simulink model "MSE452_Lab3_PMSM_ForStudent_Finalv2"  (R2023a)
settings: Solver=ode45  StartTime=0.0  StopTime=0.3  MaxStep=1e-5  RelTol=1e-3  EnableMultiTasking=on
InitFcn:
  | Idc=0;
  | Vabc=0;
  | Iw=0;
values from neighbouring files (symbols this model uses):
  Flux = 0.7213*BaseFlux    [MSE452_Lab3_parameters.m]
  Ld = 0.7029*Lb    [MSE452_Lab3_parameters.m]
  Lq = 0.7029*Lb    [MSE452_Lab3_parameters.m]
  OMEGAb_r = OMEGAb/Ppairs    (= 41.885284054)    [MSE452_Lab3_parameters.m]
  Ppairs = 8    [MSE452_Lab3_parameters.m]
  RL = 1.2 * R    [MSE452_Lab3_parameters.m]
  Rs = 0.00517*Zb    [MSE452_Lab3_parameters.m]
undefined symbols (not defined in the file or in its folder): Ts
libraries: spspowerguiLib x1
settings Model: Creator=Administrator  LastModifiedBy=mitch
settings SolverCC: ZeroCrossControl=DisableAll  AlgebraicLoopSolver=TrustRegion
settings DataIOCC: LimitDataPoints=on  SaveFormat=Array  SignalLoggingSaveFormat=ModelDataLogs  ReturnWorkspaceOutputs=off
settings OptimizationCC: BlockReduction=off  DefaultParameterBehavior=Inlined  BufferReuse=off  ExpressionDepthLimit=2147483647  InitFltsAndDblsToZero=on  LifeSpan=inf
settings DebuggingCC: SaveWithParameterizedLinksMsg=none  UnderspecifiedInitializationDetection=Classic  MergeDetectMultiDrivingBlocksExec=none  SignalResolutionControl=TryResolveAllWithWarning  SolverPrmCheckMsg=warning  MultiTaskDSMMsg=warning  MultiTaskCondExecSysMsg=none  FcnCallInpInsideContextMsg=warning  UnconnectedInputMsg=warning  UnconnectedOutputMsg=warning  UnconnectedLineMsg=warning  StateNameClashWarn=warning  SFUnexpectedBacktrackingDiag=warning  SFNoUnconditionalDefaultTransitionDiag=warning  SFExecutionAtInitializationDiag=none  ArithmeticOperatorsInVariantConditions=warning
settings HardwareCC: ProdBitPerPointer=32  ProdBitPerSizeT=32  ProdBitPerPtrDiffT=32  ProdLargestAtomicFloat=None  ProdIntDivRoundTo=Undefined  ProdEndianess=Unspecified  ProdWordSize=32  ProdHWDeviceType=32-bit Generic
settings ModelReferenceCC: PropagateSignalLabelsOutOfModel=off
settings SFSimCC: SimUseLocalCustomCode=off  CustomCodeUndefinedFunction=UseInterfaceOnly
settings RTWCC: RTWUseLocalCustomCode=off
settings CodeAppCC: StateflowObjectComments=on
settings GRTTargetCC: TargetFcnLib=ansi_tfl_tmw.mat  TargetLangStandard=C89/C90 (ANSI)  CombineOutputUpdateFcns=off  GRTInterface=on
settings ConfigComp: CovMetricSettings=dw  CovSaveCumulativeToWorkspaceVar=on  CovSaveSingleToWorkspaceVar=on  CovExternalEMLEnable=off

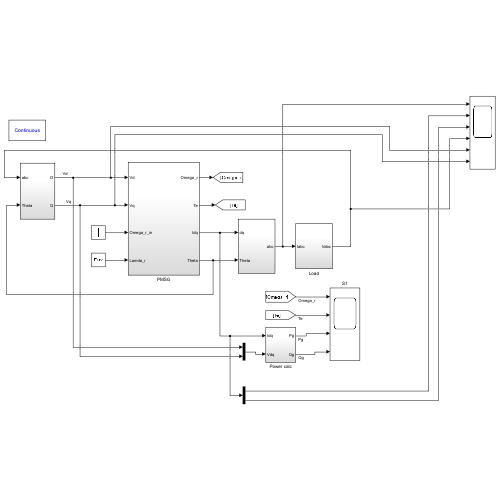
[thumbnail: Simulink's stored preview of the top-level diagram]
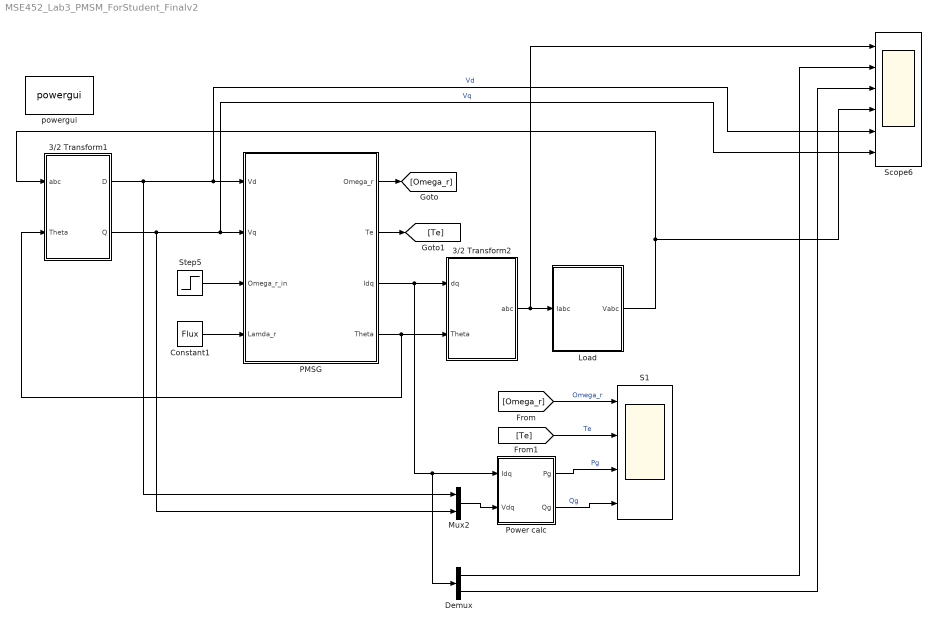
== system MSE452_Lab3_PMSM_ForStudent_Finalv2 ==
  3/2 Transform1 : Subsystem
  3/2 Transform2 : Subsystem
  Constant1 : Constant  Value=Flux
  Demux : Demux  Outputs=2
  Load : Subsystem
  Mux2 : Mux  Inputs=2
  PMSG : Subsystem
  Power calc : Subsystem
  S1 : Scope  NumInputPorts=4
  Scope6 : Scope  NumInputPorts=6
  Step5 : Step  Time=0  After=0.8*OMEGAb_r  SampleTime=0
  powergui : spspowerguiLib/powergui  SimulationMode=Continuous  SampleTime=Ts  frequency=60  Iterations=50  frequencyindice=1  Pbase=100e6  ErrMax=1e-4  UnitsV=kV  UnitsW=MW  buscounter=0  FunctionMessages=off  echomessages=off  EnableUseOfTLC=off  CurrentSourceSwitches=off  DisableSnubberDevices=off  DisableRonSwitches=off  DisableVfSwitches=off  DisplayEquations=off  AutomaticDiscreteSolvers=off  SolverType=Tustin  Interpol=off  ExternalGateDelay=off  methode=off  Ts=0  x0status=blocks  SPID=off  SwTol=0  HookPort=off  NonlinearTolerance=1e-4  nMaxIteration=100  ContinueOnMaxIteration=off  RestoreLinks=warning  ResistiveCurrentMeasurement=off  Frange=[0:2:500]  Ylog=off  Xlog=on  ShowGrid=off  save=off  variable=ZData  structure=GridVIWave  ZoomFFT=off  StartTime=2  cycles=12  DisplayStyle=1  fundamental=60  FreqAxis=on  MaxFrequency=60*15  frequencyindicesteady=1  RmsSteady=1  display=off
  wires:
  PMSG/3(Idq) -> 3/2 Transform2/1(dq), Demux/1, Power calc/1(Idq)
  3/2 Transform1/2(Q) -> Scope6/6, PMSG/2(Vq), Mux2/2  "Vq"
  3/2 Transform1/1(D) -> Scope6/5, PMSG/1(Vd), Mux2/1  "Vd"
  PMSG/1(Omega_r) -> [Omega_r]
  PMSG/2(Te) -> [Te]
  Step5/1 -> PMSG/3(Omega_r_in)
  PMSG/4(Theta) -> 3/2 Transform2/2(Theta), 3/2 Transform1/2(Theta)
  Mux2/1 -> Power calc/2(Vdq)
  Constant1/1 -> PMSG/4(Lamda_r)
  Load/1(Vabc) -> 3/2 Transform1/1(abc), Scope6/4
  Power calc/2(Qg) -> S1/4  "Qg"
  Power calc/1(Pg) -> S1/3  "Pg"
  [Omega_r] -> S1/1  "Omega_r"
  [Te] -> S1/2  "Te"
  3/2 Transform2/1(abc) -> Scope6/1, Load/1(Iabc)
  Demux/1 -> Scope6/2
  Demux/2 -> Scope6/3

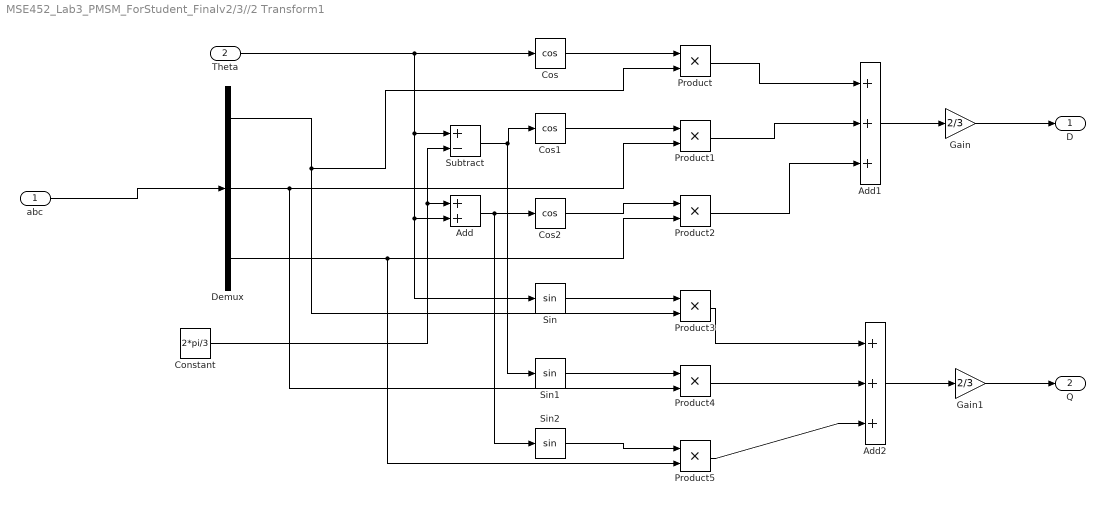
== system MSE452_Lab3_PMSM_ForStudent_Finalv2/3//2 Transform1 ==
  abc : Inport
  Theta : Inport  Port=2
  Add : Sum
  Add1 : Sum  Inputs=+++
  Add2 : Sum  Inputs=+++
  Constant : Constant  Value=2*pi/3
  Cos : Trigonometry  Operator=cos
  Cos1 : Trigonometry  Operator=cos
  Cos2 : Trigonometry  Operator=cos
  Demux : Demux  Outputs=3
  Gain : Gain  Gain=2/3
  Gain1 : Gain  Gain=2/3
  Product{,1..5} (6 alike) : Product
  Sin : Trigonometry
  Sin1 : Trigonometry
  Sin2 : Trigonometry
  Subtract : Sum  Inputs=+-
  D : Outport
  Q : Outport  Port=2
  wires:
  Theta/1 -> Sin/1, Add/2, Subtract/1, Cos/1
  Add2/1 -> Gain1/1
  Add1/1 -> Gain/1
  Product/1 -> Add1/1
  Product1/1 -> Add1/2
  Product2/1 -> Add1/3
  Product3/1 -> Add2/1
  Product4/1 -> Add2/2
  Product5/1 -> Add2/3
  Cos/1 -> Product/1
  Subtract/1 -> Sin1/1, Cos1/1
  Add/1 -> Cos2/1, Sin2/1
  Sin2/1 -> Product5/1
  Sin1/1 -> Product4/1
  Sin/1 -> Product3/1
  Cos2/1 -> Product2/1
  Cos1/1 -> Product1/1
  Constant/1 -> Subtract/2, Add/1
  Demux/2 -> Product4/2, Product1/2
  Demux/3 -> Product2/2, Product5/2
  Demux/1 -> Product/2, Product3/2
  Gain1/1 -> Q/1
  Gain/1 -> D/1
  abc/1 -> Demux/1

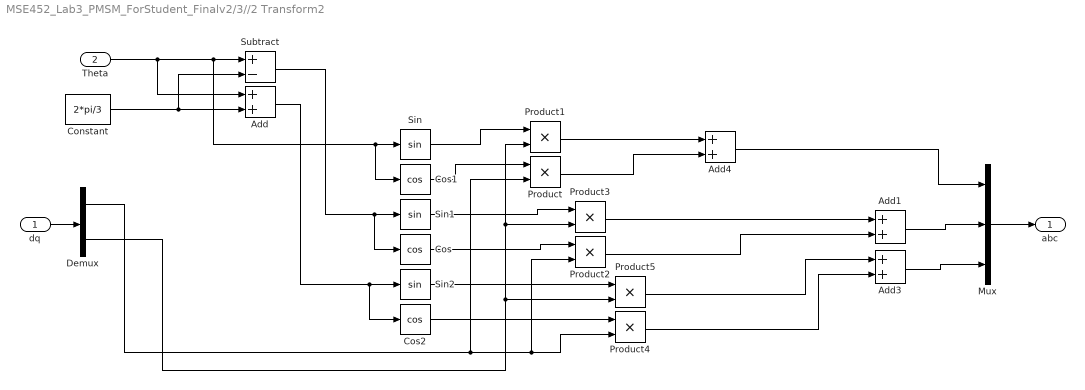
== system MSE452_Lab3_PMSM_ForStudent_Finalv2/3//2 Transform2 ==
  dq : Inport
  Theta : Inport  Port=2
  Add{,1,3..4} (4 alike) : Sum
  Constant : Constant  Value=2*pi/3  VectorParams1D=off
  Cos : Trigonometry  Operator=cos
  Cos1 : Trigonometry  Operator=cos
  Cos2 : Trigonometry  Operator=cos
  Demux : Demux  Outputs=2
  Mux : Mux  Inputs=3
  Product{,1..5} (6 alike) : Product
  Sin : Trigonometry
  Sin1 : Trigonometry
  Sin2 : Trigonometry
  Subtract : Sum  Inputs=+-
  abc : Outport
  wires:
  dq/1 -> Demux/1
  Mux/1 -> abc/1
  Add4/1 -> Mux/1
  Add1/1 -> Mux/2
  Add3/1 -> Mux/3
  Theta/1 -> Add/1, Cos1/1, Sin/1, Subtract/1
  Constant/1 -> Add/2, Subtract/2
  Subtract/1 -> Cos/1, Sin1/1
  Add/1 -> Cos2/1, Sin2/1
  Cos1/1 -> Product/1
  Sin/1 -> Product1/1
  Product1/1 -> Add4/1
  Product/1 -> Add4/2
  Product3/1 -> Add1/1
  Product2/1 -> Add1/2
  Cos/1 -> Product2/1
  Sin1/1 -> Product3/1
  Sin2/1 -> Product5/1
  Cos2/1 -> Product4/1
  Product5/1 -> Add3/1
  Product4/1 -> Add3/2
  Demux/2 -> Product5/2, Product3/2, Product1/2
  Demux/1 -> Product/2, Product2/2, Product4/2

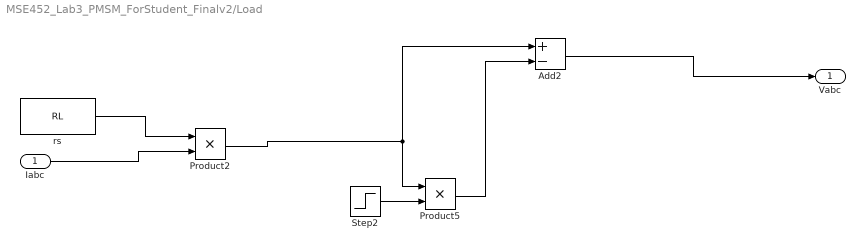
== system MSE452_Lab3_PMSM_ForStudent_Finalv2/Load ==
  Iabc : Inport
  Add2 : Sum  Inputs=+-
  Product2 : Product
  Product5 : Product
  Step2 : Step  Time=0.1  After=.5  SampleTime=0
  rs : Constant  Value=RL
  Vabc : Outport
  wires:
  Iabc/1 -> Product2/2
  rs/1 -> Product2/1
  Product2/1 -> Product5/1, Add2/1
  Step2/1 -> Product5/2
  Product5/1 -> Add2/2
  Add2/1 -> Vabc/1

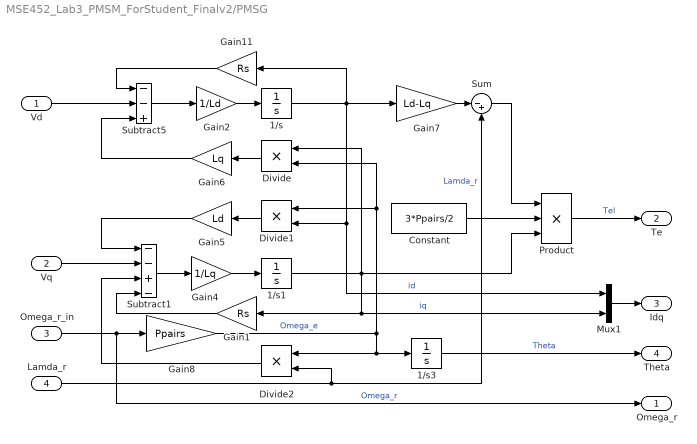
== system MSE452_Lab3_PMSM_ForStudent_Finalv2/PMSG ==
  Vd : Inport
  Vq : Inport  Port=2
  Omega_r_in : Inport  Port=3
  Lamda_r : Inport  Port=4
  1/s : Integrator
  1/s1 : Integrator
  1/s3 : Integrator
  Constant : Constant  Value=3*Ppairs/2
  Divide : Product  Inputs=**
  Divide1 : Product  Inputs=**
  Divide2 : Product  Inputs=**
  Gain1 : Gain  Gain=Rs
  Gain11 : Gain  Gain=Rs
  Gain2 : Gain  Gain=1/Ld
  Gain4 : Gain  Gain=1/Lq
  Gain5 : Gain  Gain=Ld
  Gain6 : Gain  Gain=Lq
  Gain7 : Gain  Gain=Ld-Lq
  Gain8 : Gain  Gain=Ppairs
  Mux1 : Mux  Inputs=2
  Product : Product  Inputs=3  RndMeth=Zero
  Subtract1 : Sum  Inputs=--+-
  Subtract5 : Sum  Inputs=--+
  Sum : Sum  Inputs=|-+
  Omega_r : Outport
  Te : Outport  Port=2
  Idq : Outport  Port=3
  Theta : Outport  Port=4
  wires:
  Divide2/1 -> Subtract1/3
  Product/1 -> Te/1  "Tel"
  Constant/1 -> Product/2
  Sum/1 -> Product/1
  Gain7/1 -> Sum/1
  Gain5/1 -> Subtract1/1
  Gain6/1 -> Subtract5/3
  Divide1/1 -> Gain5/1
  Divide/1 -> Gain6/1
  1/s1/1 -> Divide/1, Product/3, Mux1/2, Gain1/1  "iq"
  Gain4/1 -> 1/s1/1
  Subtract1/1 -> Gain4/1
  1/s/1 -> Divide1/2, Mux1/1, Gain7/1, Gain11/1  "id"
  Gain2/1 -> 1/s/1
  Subtract5/1 -> Gain2/1
  Vd/1 -> Subtract5/2
  Vq/1 -> Subtract1/2
  Mux1/1 -> Idq/1
  Gain11/1 -> Subtract5/1
  Lamda_r/1 -> Divide2/2, Sum/2  "Lamda_r"
  Omega_r_in/1 -> Gain8/1, Omega_r/1  "Omega_r"
  1/s3/1 -> Theta/1  "Theta"
  Gain1/1 -> Subtract1/4
  Gain8/1 -> Divide1/1, Divide/2, Divide2/1, 1/s3/1  "Omega_e"

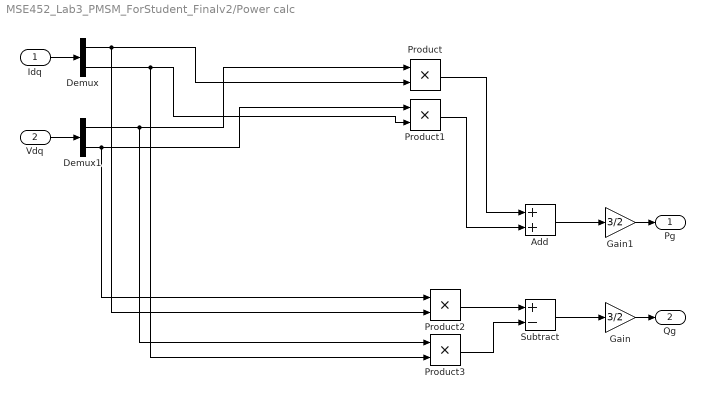
== system MSE452_Lab3_PMSM_ForStudent_Finalv2/Power calc ==
  Idq : Inport
  Vdq : Inport  Port=2
  Add : Sum
  Demux : Demux  Outputs=2
  Demux1 : Demux  Outputs=2
  Gain : Gain  Gain=3/2
  Gain1 : Gain  Gain=3/2
  Product{,1..3} (4 alike) : Product
  Subtract : Sum  Inputs=+-
  Pg : Outport
  Qg : Outport  Port=2
  wires:
  Add/1 -> Gain1/1
  Subtract/1 -> Gain/1
  Demux1/1 -> Product3/1, Product/1
  Demux1/2 -> Product2/1, Product1/1
  Demux/1 -> Product2/2, Product/2
  Demux/2 -> Product1/2, Product3/2
  Product/1 -> Add/1
  Product1/1 -> Add/2
  Product2/1 -> Subtract/1
  Product3/1 -> Subtract/2
  Gain1/1 -> Pg/1
  Gain/1 -> Qg/1
  Idq/1 -> Demux/1
  Vdq/1 -> Demux1/1
